simulink model "MassSpringDamperModelEvents"  (R2026a)
settings: Solver=VariableStepAuto  StopTime=20  MaxStep=inf  RelTol=1e-6
model workspace (MAT data in the model file):
  b = 3
  k = 128
  m = 2
  x0 = 0.5
Description:
  | The van der Pol Equation
  | 
  | This is a simulation of a nonlinear second order system.
settings Model: ExtModeAutoUpdateStatusClock=off  Creator=The MathWorks, Inc.  LastModifiedBy=kdeeley
settings DataIOCC: ExternalInput=[]  InitialState=[]  TimeSaveName=t  OutputSaveName=y
settings OptimizationCC: BooleanDataType=off  InitFltsAndDblsToZero=on  BufferReusableBoundary=off
settings DebuggingCC: SaveWithParameterizedLinksMsg=none  SignalResolutionControl=TryResolveAllWithWarning  MultiTaskDSMMsg=warning  MultiTaskCondExecSysMsg=none  BusObjectLabelMismatch=none  PregeneratedLibrarySubsystemCodeDiagnostic=none
settings HardwareCC: ProdHWDeviceType=32-bit Generic  TargetUnknown=on
settings GRTTargetCC: TargetFcnLib=ansi_tfl_tmw.mat  CombineOutputUpdateFcns=off  GRTInterface=on

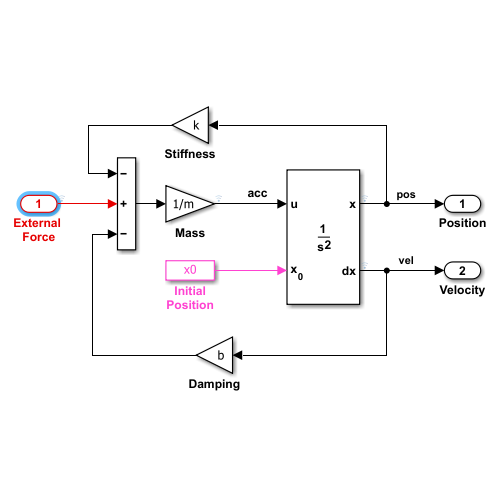
[thumbnail: Simulink's stored preview of the top-level diagram]
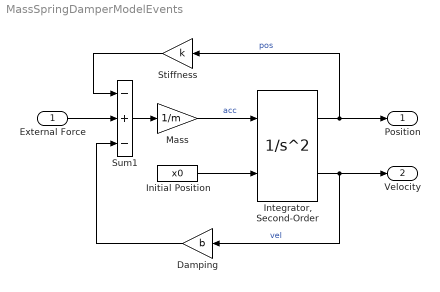
== system MassSpringDamperModelEvents ==
  External Force : Inport  SampleTime=1  Interpolate=off
  Damping : Gain  Gain=b
  Initial Position : Constant  Value=x0
  "Integrator, Second-Order" : SecondOrderIntegrator  ICSourceX=external  StateNameX='pos'  StateNameDXDT='vel'  ReinitDXDTwhenXreachesSaturation=on
  Mass : Gain  Gain=1/m
  Stiffness : Gain  Gain=k
  Sum1 : Sum  Inputs=-+-
  Position : Outport  VectorParamsAs1DForOutWhenUnconnected=off
  Velocity : Outport  Port=2  VectorParamsAs1DForOutWhenUnconnected=off
  wires:
  Sum1/1 -> Mass/1
  Mass/1 -> "Integrator, Second-Order"/1  "acc"
  External Force/1 -> Sum1/2
  "Integrator, Second-Order"/1 -> Stiffness/1, Position/1  "pos"
  Stiffness/1 -> Sum1/1
  "Integrator, Second-Order"/2 -> Damping/1, Velocity/1  "vel"
  Initial Position/1 -> "Integrator, Second-Order"/2
  Damping/1 -> Sum1/3
